simulink model "Bsw_PMSMCtrl_SimInput"  (R2023a)
settings: Solver=FixedStepDiscrete  StartTime=0.0  StopTime=0.3  RelTol=1e-3
PreLoadFcn:
  | addpath("Sim\")
  | Sim_PreLoad_PMSMCtrl;
settings Model: Creator=62555  LastModifiedBy=62555
settings OptimizationCC: DefaultParameterBehavior=Inlined  UseDivisionForNetSlopeComputation=on  DefaultUnderspecifiedDataType=single  EnhancedBackFolding=on  PassReuseOutputArgsAs=Individual arguments  ZeroExternalMemoryAtStartup=off  ZeroInternalMemoryAtStartup=off  OptimizeBlockOrder=speed  DifferentSizesBufferReuse=on  OptimizationCustomize=off  EfficientTunableParamExpr=on
settings DebuggingCC: ParameterTunabilityLossMsg=error
settings SFSimCC: MATLABDynamicMemAlloc=off
settings RTWCC: Description=Embedded Coder  SystemTargetFile=ert.tlc  GenCodeOnly=on  TemplateMakefile=ert_default_tmf  GenerateReport=on  LaunchReport=on
settings CodeAppCC: ForceParamTrailComments=on  IgnoreCustomStorageClasses=off  OperatorAnnotations=on  SimulinkDataObjDesc=on  SFDataObjDesc=on  InsertBlockDesc=on
settings ERTTargetCC: TargetLangStandard=C99 (ISO)  GenerateSampleERTMain=on  InlinedParameterPlacement=NonHierarchical  ERTCustomFileTemplate=example_file_process.tlc

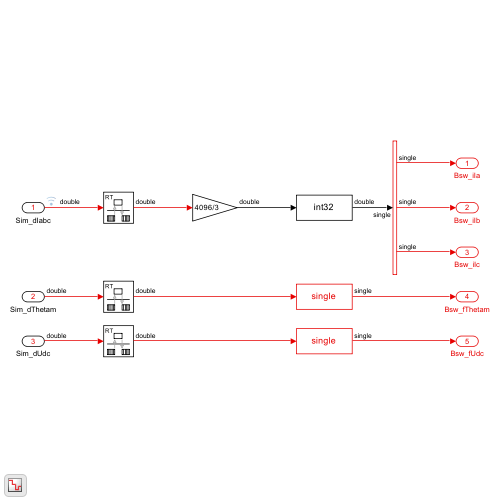
[thumbnail: Simulink's stored preview of the top-level diagram]
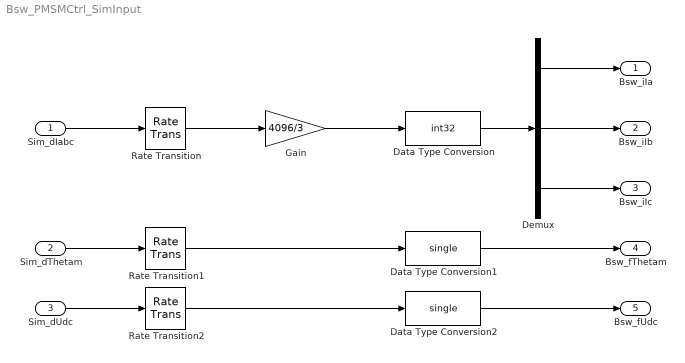
== system Bsw_PMSMCtrl_SimInput ==
  Sim_dIabc : Inport  OutDataTypeStr=double
  Sim_dThetam : Inport  Port=2  OutDataTypeStr=double
  Sim_dUdc : Inport  Port=3  OutDataTypeStr=double
  Data Type Conversion : DataTypeConversion  OutDataTypeStr=int32  SaturateOnIntegerOverflow=off  RndMeth=Floor
  Data Type Conversion1 : DataTypeConversion  OutDataTypeStr=single  SaturateOnIntegerOverflow=off  RndMeth=Floor
  Data Type Conversion2 : DataTypeConversion  OutDataTypeStr=single  SaturateOnIntegerOverflow=off  RndMeth=Floor
  Demux : Demux  Outputs=3
  Gain : Gain  Gain=4096/3
  Rate Transition : RateTransition  OutPortSampleTime=Sw_Par_fTs
  Rate Transition1 : RateTransition  OutPortSampleTime=Sw_Par_fTs
  Rate Transition2 : RateTransition  OutPortSampleTime=Sw_Par_fTs
  Bsw_iIa : Outport
  Bsw_iIb : Outport  Port=2
  Bsw_iIc : Outport  Port=3
  Bsw_fThetam : Outport  Port=4
  Bsw_fUdc : Outport  Port=5
  wires:
  Data Type Conversion2/1 -> Bsw_fUdc/1
  Rate Transition2/1 -> Data Type Conversion2/1
  Rate Transition1/1 -> Data Type Conversion1/1
  Demux/2 -> Bsw_iIb/1
  Data Type Conversion1/1 -> Bsw_fThetam/1
  Rate Transition/1 -> Gain/1
  Demux/1 -> Bsw_iIa/1
  Sim_dThetam/1 -> Rate Transition1/1
  Sim_dUdc/1 -> Rate Transition2/1
  Demux/3 -> Bsw_iIc/1
  Sim_dIabc/1 -> Rate Transition/1
  Gain/1 -> Data Type Conversion/1
  Data Type Conversion/1 -> Demux/1
